simulink model "QpskEqualization"  (R2015a)
settings: Solver=ode45  StartTime=0.0  StopTime=Inf  RelTol=1e-3
undefined symbols (not defined in the file): j
libraries: commdigbbndpm3 x2, commsink2 x1, commchan3 x1, commrandsrc2 x1, commeq2 x1
settings Model: Creator=konstantis  LastModifiedBy=konstantis

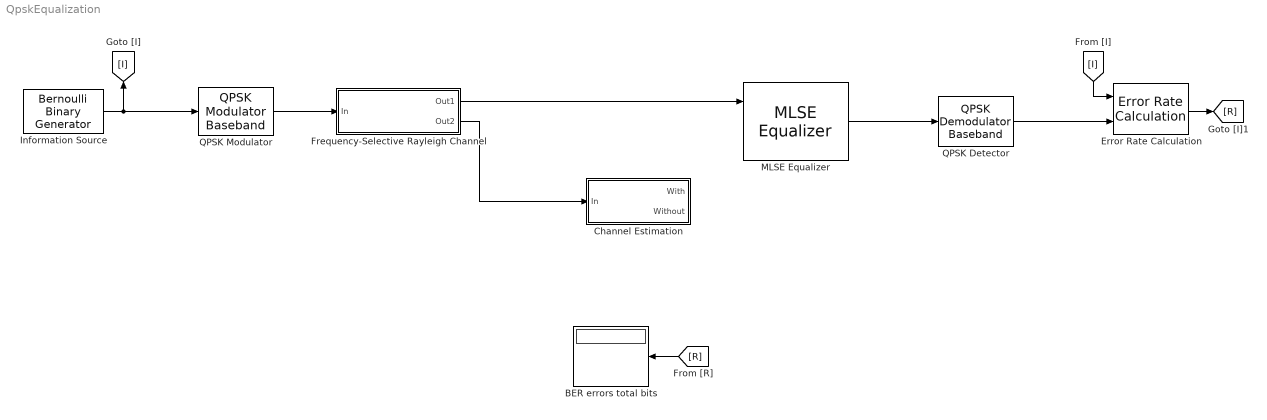
== system QpskEqualization ==
  BER errors total bits : Display
      settings: Format=short_e
  Channel Estimation : Subsystem
  Error Rate Calculation : commsink2/Error Rate Calculation  N=0  st_delay=0  cp_mode=Entire frame  subframe=[]  PMode=Port  WsName=ErrorVec  RsMode2=off  stop=off  numErr=100  maxBits=1e6
  Frequency-Selective Rayleigh Channel : Subsystem
  Information Source : commrandsrc2/Bernoulli Binary Generator  P=0.5  seed=61  Ts=.001  frameBased=on  sampPerFrame=1000  orient=off  outDataType=double
  MLSE Equalizer : commeq2/MLSE Equalizer  specchan=Input port  chancoeff=[1 1 1]'  constpts=[1+j -1+j -1-j 1-j]*sqrt(2)/2  tbdepth=500  opmode=Reset every frame  enpreamble=off  preamble=[0 3 2 1]  enpostamble=off  postamble=[0 2 3 1]  numsamp=1  reset=off
  QPSK Detector : commdigbbndpm3/QPSK Demodulator Baseband  Ph=pi/4  Dec=Gray  OutType=Bit  DecType=Hard decision  VarSource=Dialog  Variance=1  outDtype1=Inherit via internal rule  outDtype2=Inherit via internal rule  derotateFactorWordLen=16
  QPSK Modulator : commdigbbndpm3/QPSK Modulator Baseband  InType=Bit  Enc=Gray  Ph=pi/4  outDtype=double  outWordLen=16  outUDDataType=sfix(16)  outFracLenMode=Best precision  outFracLen=15
  wires:
  Information Source/1 -> QPSK Modulator/1, [I]
  MLSE Equalizer/1 -> QPSK Detector/1
  QPSK Detector/1 -> Error Rate Calculation/2
  QPSK Modulator/1 -> Frequency-Selective Rayleigh Channel/1(In)
  Frequency-Selective Rayleigh Channel/1(Out1) -> MLSE Equalizer/1
  Frequency-Selective Rayleigh Channel/2(Out2) -> Channel Estimation/1(In)
  [I] -> Error Rate Calculation/1
  Error Rate Calculation/1 -> [R]
  [R] -> BER errors total bits/1

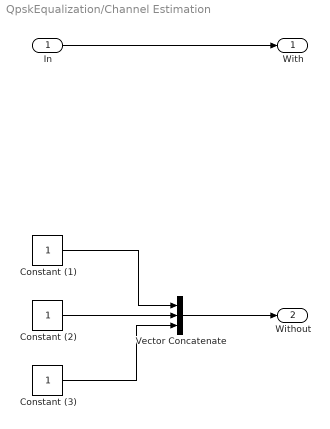
== system QpskEqualization/Channel Estimation ==
  In : Inport
  Constant (1) : Constant
  Constant (2) : Constant
  Constant (3) : Constant
  Vector Concatenate : Concatenate  NumInputs=3
  With : Outport
  Without : Outport  Port=2
  wires:
  In/1 -> With/1
  Vector Concatenate/1 -> Without/1
  Constant (1)/1 -> Vector Concatenate/1
  Constant (2)/1 -> Vector Concatenate/2
  Constant (3)/1 -> Vector Concatenate/3

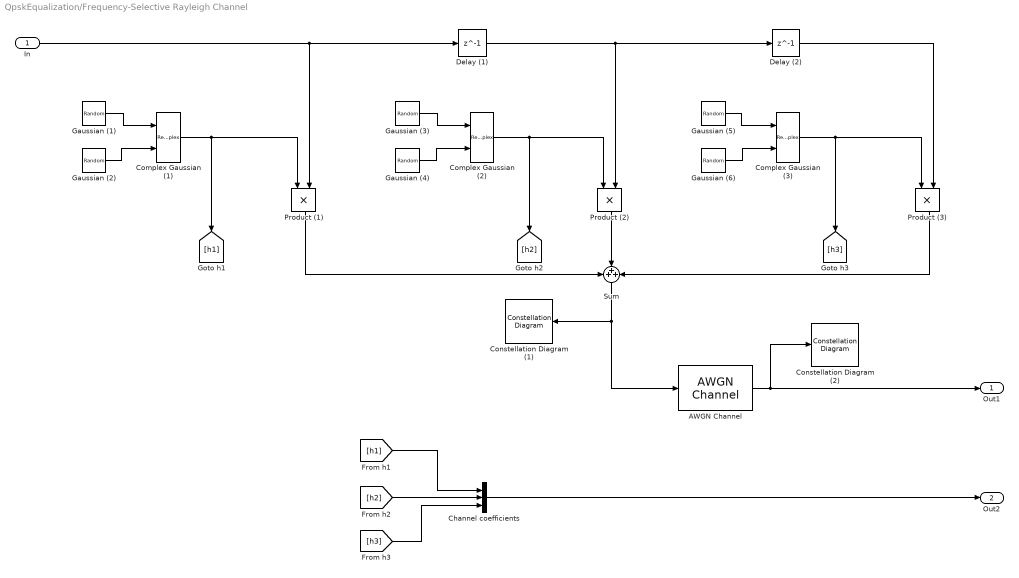
== system QpskEqualization/Frequency-Selective Rayleigh Channel ==
  In : Inport
  AWGN Channel : commchan3/AWGN Channel  InputProcessing=Columns as channels (frame based)  seed=67  noiseMode="Signal to noise ratio  (SNR)"  EbNodB=14  EsNodB=20  SNRdB=40  bitsPerSym=2  Ps=1  Tsym=.002  variance=1
  Channel coefficients : Concatenate  NumInputs=3
  Complex Gaussian (1) : RealImagToComplex
  Complex Gaussian (2) : RealImagToComplex
  Complex Gaussian (3) : RealImagToComplex
  Constellation Diagram (1) : ConstellationDiagram
  Constellation Diagram (2) : ConstellationDiagram
  Delay (1) : Delay  DelayLength=1  InitialCondition=0  InputProcessing=Columns as channels (frame based)  SampleTime=1
  Delay (2) : Delay  DelayLength=1  InitialCondition=0  InputProcessing=Columns as channels (frame based)  SampleTime=1
  Gaussian (1) : RandomNumber  Variance=1/6  SampleTime=1
  Gaussian (2) : RandomNumber  Variance=1/6  Seed=2^30  SampleTime=1
  Gaussian (3) : RandomNumber  Variance=1/6  Seed=2^31  SampleTime=1
  Gaussian (4) : RandomNumber  Variance=1/6  Seed=2^32  SampleTime=1
  Gaussian (5) : RandomNumber  Variance=1/6  Seed=2^33  SampleTime=1
  Gaussian (6) : RandomNumber  Variance=1/6  Seed=2^34  SampleTime=1
  Product (1) : Product
  Product (2) : Product
  Product (3) : Product
  Sum : Sum  Inputs=+++
  Out1 : Outport
  Out2 : Outport  Port=2
  wires:
  In/1 -> Product (1)/2, Delay (1)/1
  Delay (1)/1 -> Delay (2)/1, Product (2)/2
  Delay (2)/1 -> Product (3)/2
  Product (1)/1 -> Sum/1
  Product (2)/1 -> Sum/2
  Product (3)/1 -> Sum/3
  Gaussian (1)/1 -> Complex Gaussian (1)/1
  Gaussian (2)/1 -> Complex Gaussian (1)/2
  Gaussian (3)/1 -> Complex Gaussian (2)/1
  Gaussian (4)/1 -> Complex Gaussian (2)/2
  Gaussian (5)/1 -> Complex Gaussian (3)/1
  Gaussian (6)/1 -> Complex Gaussian (3)/2
  Complex Gaussian (1)/1 -> Product (1)/1, [h1]
  Complex Gaussian (2)/1 -> Product (2)/1, [h2]
  Complex Gaussian (3)/1 -> Product (3)/1, [h3]
  Sum/1 -> Constellation Diagram (1)/1, AWGN Channel/1
  AWGN Channel/1 -> Out1/1, Constellation Diagram (2)/1
  [h1] -> Channel coefficients/1
  [h2] -> Channel coefficients/2
  [h3] -> Channel coefficients/3
  Channel coefficients/1 -> Out2/1
